simulink subsystem "StudentTemplate_minimal"  (R2026a)
settings: Solver=VariableStepAuto
InitFcn:
  | simstruct_init(0);
StartFcn:
  | proj_root = fileparts(fileparts(fileparts(which('launch_virtual_testbed.m')))); fid = fopen(fullfile(proj_root, 'firmware', 'build', 'matlab_callbacks.log'), 'a'); if fid ~= -1, fprintf(fid, '%s: StartFcn triggered\n', datestr(now)); fclose(fid); end; run(which('launch_virtual_testbed.m'));
StopFcn:
  | proj_root = fileparts(fileparts(fileparts(which('launch_virtual_testbed.m')))); fid = fopen(fullfile(proj_root, 'firmware', 'build', 'matlab_callbacks.log'), 'a'); if fid ~= -1, fprintf(fid, '%s: StopFcn triggered\n', datestr(now)); fclose(fid); end; clear mex; clear functions; if ~ispc, [~, ~] = system('/usr/bin/pkill -f ''[p]hysics_sim.py'' '); else, [~, ~] = system('powershell -Command \"Get-CimInstance Win32_Process -Filter \\\"CommandLine like ''%physics_sim.py%''\\\" | Invoke-CimMethod -MethodName Terminate\" >nul 2>&1'); end
libraries: simulink x1
settings Model: Creator=JesseJabezArendse  LastModifiedBy=vince
settings SFSimCC: SimUserLibraries=C:\ProgramData\MATLAB\SupportPackages\R2026a\3P.instrset\mingw_w64.instrset\x86_64-w64-mingw32\lib\libws2_32.a
settings RTWCC: PostCodeGenCommand=flash_micromouse(buildInfo)

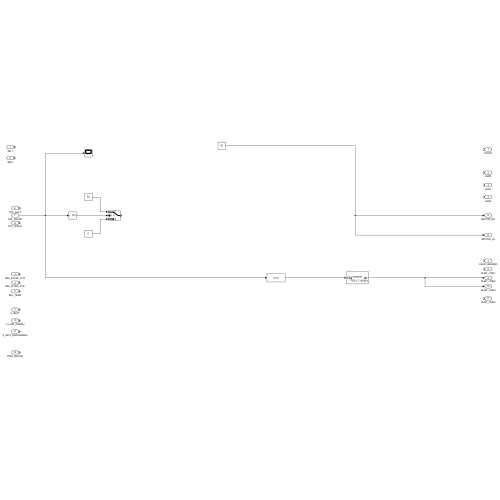
[thumbnail: Simulink's stored preview of the top-level diagram]
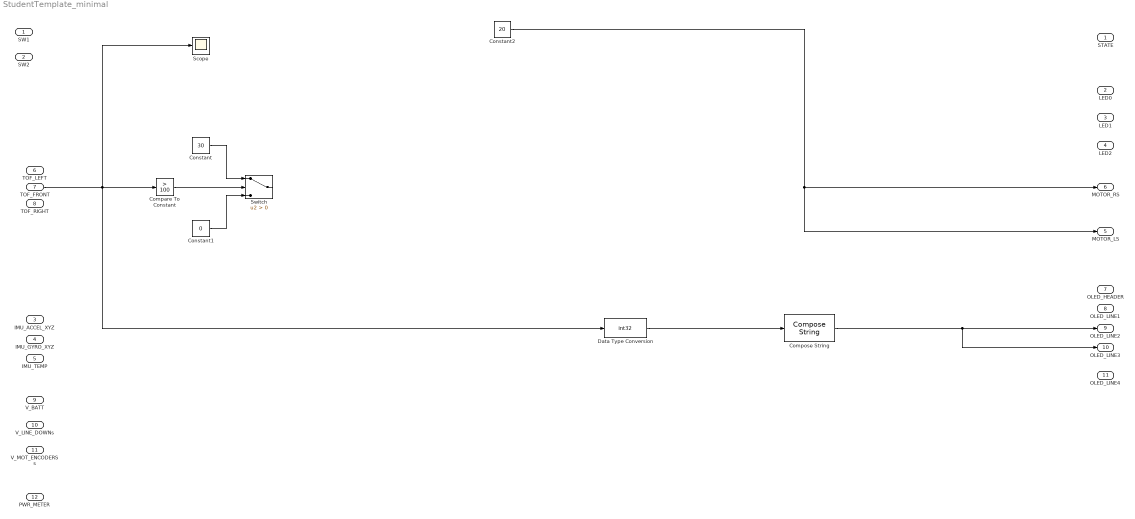
== system StudentTemplate_minimal ==
  SW1 : Inport
  SW2 : Inport  Port=2
  IMU_ACCEL_XYZ : Inport  Port=3
  IMU_GYRO_XYZ : Inport  Port=4
  IMU_TEMP : Inport  Port=5
  TOF_LEFT : Inport  Port=6
  TOF_FRONT : Inport  Port=7
  TOF_RIGHT : Inport  Port=8
  V_BATT : Inport  Port=9
  V_LINE_DOWNs : Inport  Port=10
  V_MOT_ENCODERSs : Inport  Port=11
  PWR_METER : Inport  Port=12
  Compare To Constant : simulink/Logic and Bit Operations/Compare To Constant  relop=>  const=100  OutDataTypeStr=boolean
  Compose String : ComposeString  Format="\"TOF_C: %03d mm\""
  Constant : Constant  Value=30
  Constant1 : Constant  Value=0
  Constant2 : Constant  Value=20
  Data Type Conversion : DataTypeConversion  OutDataTypeStr=int32  SaturateOnIntegerOverflow=off  RndMeth=Floor
  Scope : Scope
      settings: ActiveDisplayYMinimum=-1  ActiveDisplayYMaximum=1
  Switch : Switch  Criteria=u2 > Threshold  SaturateOnIntegerOverflow=off  InputSameDT=off
  STATE : Outport
  LED0 : Outport  Port=2
  LED1 : Outport  Port=3
  LED2 : Outport  Port=4
  MOTOR_LS : Outport  Port=5
  MOTOR_RS : Outport  Port=6
  OLED_HEADER : Outport  Port=7
  OLED_LINE1 : Outport  Port=8
  OLED_LINE2 : Outport  Port=9
  OLED_LINE3 : Outport  Port=10
  OLED_LINE4 : Outport  Port=11
  wires:
  Compare To Constant/1 -> Switch/2
  Constant/1 -> Switch/1
  Constant1/1 -> Switch/3
  TOF_FRONT/1 -> Compare To Constant/1, Data Type Conversion/1, Scope/1
  Data Type Conversion/1 -> Compose String/1
  Compose String/1 -> OLED_LINE3/1, OLED_LINE2/1
  Constant2/1 -> MOTOR_RS/1, MOTOR_LS/1
